simulink model "tarefa6"  (R2022b)
settings: Solver=VariableStepAuto  StartTime=0.0  StopTime=30  RelTol=1e-3
values from neighbouring files (symbols this model uses):
  Cd = ss_d.C    [lab6.m]
  d = -0.15    [lab6.m]
  Dd = ss_d.D    [lab6.m]
  F = ss_d.A    [lab6.m]
  H = ss_d.B    [lab6.m]
  R = 1.25    [lab6.m]
  td = 15    [lab6.m]
undefined symbols (not defined in the file or in its folder): Ac, Bc, Cc, Dc
settings Model: Creator=hugo_  LastModifiedBy=hugo_

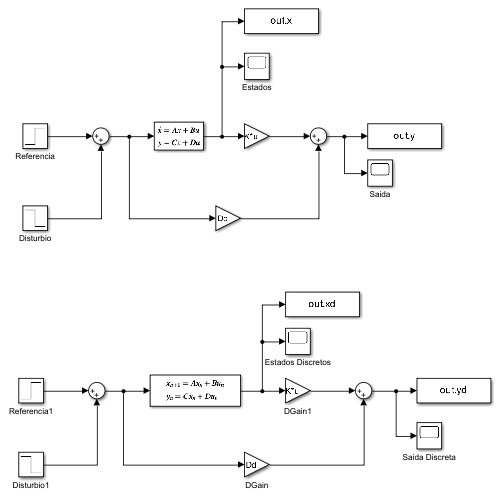
[thumbnail: Simulink's stored preview of the top-level diagram]
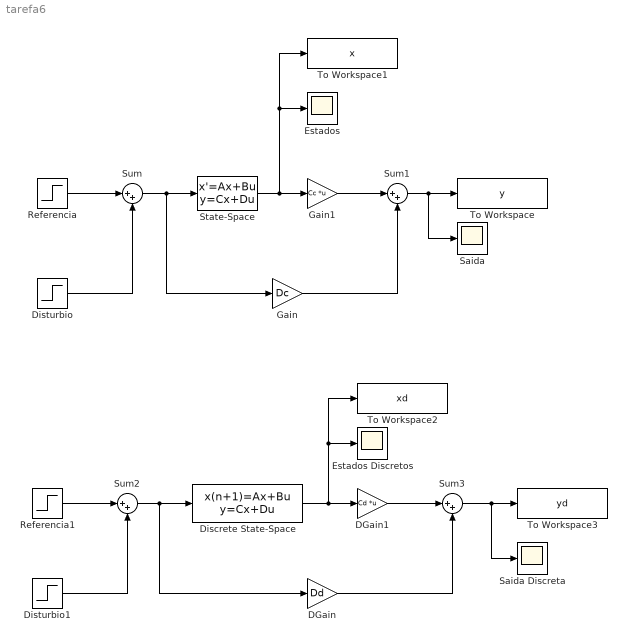
== system tarefa6 ==
  DGain : Gain  Gain=Dd
  DGain1 : Gain  Gain=Cd  Multiplication=Matrix(K*u)
  Discrete State-Space : DiscreteStateSpace  A=F  B=H  C=[1 0; 0 1]  D=[0;0]  SampleTime=-1
  Disturbio : Step  Time=td  After=d  SampleTime=0
  Disturbio1 : Step  Time=td  After=d  SampleTime=0
  Estados : Scope
  Estados Discretos : Scope
  Gain : Gain  Gain=Dc
  Gain1 : Gain  Gain=Cc  Multiplication=Matrix(K*u)
  Referencia : Step  Time=0  After=R  SampleTime=0
  Referencia1 : Step  Time=0  After=R  SampleTime=0
  Saida : Scope
  Saida Discreta : Scope
  State-Space : StateSpace  A=Ac  B=Bc  C=[1 0; 0 1]  D=[0;0]  InitialCondition=0  ParameterTunability=Unconstrained
  Sum{,1..3} (4 alike) : Sum  Inputs=|++
  To Workspace : ToWorkspace  VariableName=y  SaveFormat=Timeseries  SampleTime=-1
  To Workspace1 : ToWorkspace  VariableName=x  SaveFormat=Timeseries  SampleTime=-1
  To Workspace2 : ToWorkspace  VariableName=xd  SaveFormat=Timeseries  SampleTime=-1
  To Workspace3 : ToWorkspace  VariableName=yd  SaveFormat=Timeseries  SampleTime=-1
  wires:
  Referencia/1 -> Sum/1
  Disturbio/1 -> Sum/2
  Sum/1 -> Gain/1, State-Space/1
  State-Space/1 -> Estados/1, To Workspace1/1, Gain1/1
  Gain1/1 -> Sum1/1
  Gain/1 -> Sum1/2
  Sum1/1 -> Saida/1, To Workspace/1
  Referencia1/1 -> Sum2/1
  Disturbio1/1 -> Sum2/2
  Sum2/1 -> DGain/1, Discrete State-Space/1
  Discrete State-Space/1 -> To Workspace2/1, Estados Discretos/1, DGain1/1
  DGain1/1 -> Sum3/1
  Sum3/1 -> Saida Discreta/1, To Workspace3/1
  DGain/1 -> Sum3/2
